simulink model "ICAES_R2025aa_real_a"  (R2025a)
settings: Solver=FixedStepAuto  StartTime=0.0  StopTime=stopt  FixedStep=deltat  MaxStep=0.05  RelTol=1e-3
InitFcn:
  | clear all;
  | close all;
  | clc;
  | 
  | % add the data and script directories
  | addpath('data','scripts');
  | 
  | % load the constants (units)
  | constants;
  | 
  | % load the simulation parameters
  | preprocessing;
StopFcn:
  | postprocessing;
values from neighbouring files (symbols this model uses):
  c_p = 1005    [icaes_parameter_sweep.m]    (also in preprocessing.m = 1005 * unit("J") / (unit("kg") * unit("K")))
  c_tes = 4184    [icaes_parameter_sweep.m]    (also in preprocessing.m = 4184 * unit("J") / (unit("kg") * unit("K")))
  eta_comp = 0.833    [icaes_parameter_sweep.m]    (also in preprocessing.m)
  eta_exp = 0.85    [icaes_parameter_sweep.m]    (also in preprocessing.m)
  m_tes = m_tes_range(im)    [icaes_parameter_sweep.m]    (also in preprocessing.m = 5000000 * unit("kg"))
  n_poly = 1.1    [icaes_parameter_sweep.m]    (also in preprocessing.m)
  p_amb = 101325    [icaes_parameter_sweep.m]    (also in preprocessing.m = 101325 * unit("Pa"))
  P_limit = 300e6    (= 300000000)    [icaes_parameter_sweep.m]    (also in preprocessing.m = 300 * unit("MW"))
  p_store_max = 100e5    (= 10000000)    [icaes_parameter_sweep.m]    (also in preprocessing.m = 80 * unit("bar"))
  R_air = 287.05    [icaes_parameter_sweep.m]    (also in preprocessing.m = 287.05 * unit("J") / (unit("kg") * unit("K")))
  T_amb = 300    [icaes_parameter_sweep.m]    (also in preprocessing.m = 300 * unit("K"))
  T_tes_initial = T_amb    [preprocessing.m]
  V_cavern = V_cav_range(iv)    [icaes_parameter_sweep.m]    (also in preprocessing.m = 310000 * unit("m^3"))
undefined symbols (not defined in the file or in its folder): Cablelength, Cablevoltage, m_air_initial, m_air_max, mdot_max, Rprime, T_expand, T_tes_max
settings Model: Creator=joche  LastModifiedBy=ASUS
settings DataIOCC: SaveFormat=Array  SaveOutput=off  ReturnWorkspaceOutputs=off
settings OptimizationCC: ReuseModelBlockBuffer=off
settings ModelReferenceCC: EnableRefExpFcnMdlSchedulingChecks=on
settings RTWCC: GPUComputeCapability=3.5

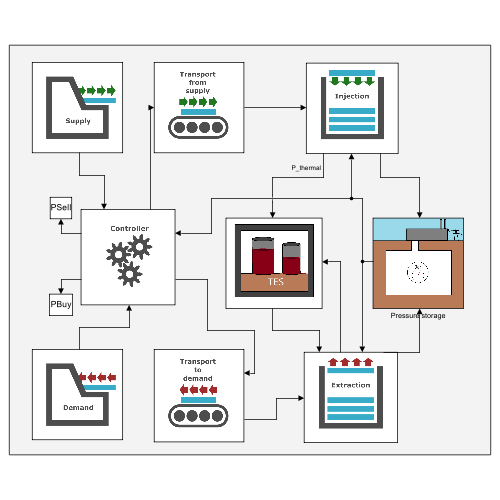
[thumbnail: Simulink's stored preview of the top-level diagram]
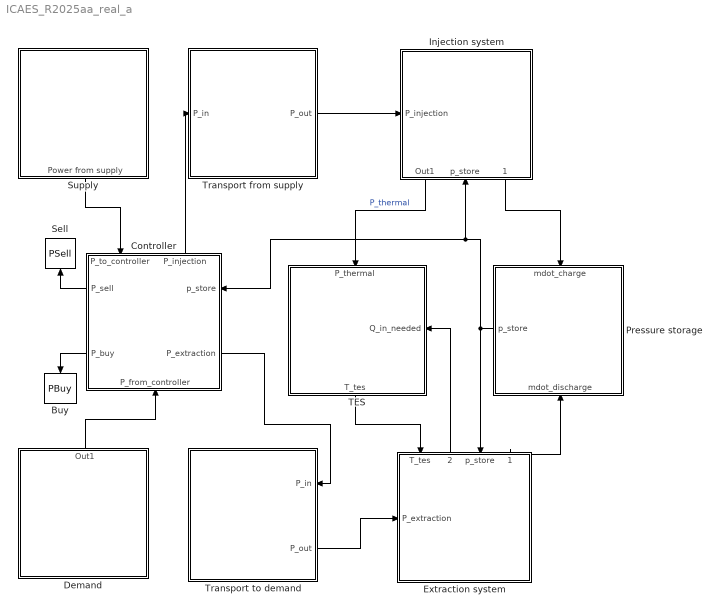
== system ICAES_R2025aa_real_a ==
  Buy : ToWorkspace  VariableName=PBuy  SampleTime=-1
  Controller : Subsystem
      settings: PortSchema="{\"entries\":[{\"content\":{\"sides\":[{\"content\":{\"connectorIds\":[\"Out3\",\"Out4\"]},\"type\":\"ConnectorPlacement.EquallySpacedRectSide\",\"uuid\":\"4daf33ce-c96a-4783-b5c4-228eed953e01\"},{\"content\":{\"connectorIds\":[\"In3\",\"Out1\"],\"side\":\"RIGHT\"},\"type\":\"ConnectorPlacement.EquallySpacedRectSide\",\"uuid\":\"e9942e50-8467-4af8-b79b-80636cbc76e5\"},{\"content\":{\"connectorIds\":[\"In1\",\"Out2\"],\"side\":\"TOP\"},\"type\":\"ConnectorPlacement.EquallySpacedRectSide\",\"uuid\":\"f315e931-d69b-4751-b712-f89c6c81baeb\"},{\"content\":{\"connectorIds\":[\"In2\"],\"side\":\"BOTTOM\"},\"type\":\"ConnectorPlacement.EquallySpacedRectSide\",\"uuid\":\"44715ee6-5cd5-4669-bcb9-5ed7c869bdb3\"}]},\"type\":\"ConnectorPlacement.EquallySpacedConnector\",\"uuid\":\"fff48899-944b-4064-b7d7-ecc12144fb48\"}],\"packageUris\":[\"http://schema.mathworks.com/mf0/Connector/R2020b\"],\"version\":\"1.0\"}"
      mask Display: image('$imagefile'); % Use "Edit Image" on toolstrip to change.
  Demand : Subsystem
      settings: PortSchema="{\"entries\":[{\"content\":{\"sides\":[{\"content\":{},\"type\":\"ConnectorPlacement.EquallySpacedRectSide\",\"uuid\":\"f27962e9-c4d7-4452-9990-e0f79d5e43d2\"},{\"content\":{\"side\":\"RIGHT\"},\"type\":\"ConnectorPlacement.EquallySpacedRectSide\",\"uuid\":\"2b278ec5-7432-4b51-af5a-f36413392bbe\"},{\"content\":{\"connectorIds\":[\"Out1\"],\"side\":\"TOP\"},\"type\":\"ConnectorPlacement.EquallySpacedRectSide\",\"uuid\":\"4ad1aacd-5412-446e-ba31-db0d1d02529a\"}]},\"type\":\"ConnectorPlacement.EquallySpacedConnector\",\"uuid\":\"5190d484-8789-4ab4-af36-e8ecab949163\"}],\"packageUris\":[\"http://schema.mathworks.com/mf0/Connector/R2020b\"],\"version\":\"1.0\"}"
      mask Display: image('$imagefile'); % Use "Edit Image" on toolstrip to change.
  Extraction system : Subsystem
      settings: PortSchema="{\"entries\":[{\"content\":{\"sides\":[{\"content\":{},\"type\":\"ConnectorPlacement.EquallySpacedRectSide\",\"uuid\":\"05c5933d-55fc-4e06-853f-fc26d42905f9\"},{\"content\":{\"connectorIds\":[\"In3\"],\"side\":\"RIGHT\"},\"type\":\"ConnectorPlacement.EquallySpacedRectSide\",\"uuid\":\"327426c5-31d5-498b-a2bd-83e49353408c\"},{\"content\":{\"side\":\"TOP\"},\"type\":\"ConnectorPlacement.EquallySpacedRectSide\",\"uuid\":\"55306cf3-a3de-4385-a5ae-b8600ecdd5a2\"},{\"content\":{\"connectorIds\":[\"Out1\",\"In1\",\"Out2\",\"In2\"],\"side\":\"BOTTOM\"},\"type\":\"ConnectorPlacement.EquallySpacedRectSide\",\"uuid\":\"08fcc9c3-40d3-4ac6-b914-dfeef6039ffb\"}]},\"type\":\"ConnectorPlacement.EquallySpacedConnector\",\"uuid\":\"cb35d5ba-e8c6-462c-b7b2-fe8356d4b0a1\"}],\"packageUris\":[\"http://schema.mathworks.com/mf0/Connector/R2020b\"],\"version\":\"1.0\"}"
      mask Display: image('$imagefile'); % Use "Edit Image" on toolstrip to change.
  Injection system : Subsystem
      settings: PortSchema="{\"entries\":[{\"content\":{\"sides\":[{\"content\":{},\"type\":\"ConnectorPlacement.EquallySpacedRectSide\",\"uuid\":\"05c5933d-55fc-4e06-853f-fc26d42905f9\"},{\"content\":{\"connectorIds\":[\"In2\"],\"side\":\"RIGHT\"},\"type\":\"ConnectorPlacement.EquallySpacedRectSide\",\"uuid\":\"327426c5-31d5-498b-a2bd-83e49353408c\"},{\"content\":{\"connectorIds\":[\"Out1\",\"In1\",\"Out2\"],\"side\":\"TOP\"},\"type\":\"ConnectorPlacement.EquallySpacedRectSide\",\"uuid\":\"55306cf3-a3de-4385-a5ae-b8600ecdd5a2\"},{\"content\":{\"side\":\"BOTTOM\"},\"type\":\"ConnectorPlacement.EquallySpacedRectSide\",\"uuid\":\"08fcc9c3-40d3-4ac6-b914-dfeef6039ffb\"}]},\"type\":\"ConnectorPlacement.EquallySpacedConnector\",\"uuid\":\"cb35d5ba-e8c6-462c-b7b2-fe8356d4b0a1\"}],\"packageUris\":[\"http://schema.mathworks.com/mf0/Connector/R2020b\"],\"version\":\"1.0\"}"
      mask Display: image('$imagefile'); % Use "Edit Image" on toolstrip to change.
  Pressure storage : Subsystem
      settings: PortSchema="{\"entries\":[{\"content\":{\"sides\":[{\"content\":{\"connectorIds\":[\"Out1\"]},\"type\":\"ConnectorPlacement.EquallySpacedRectSide\",\"uuid\":\"d889665d-bfbe-4c74-9411-d83433156a63\"},{\"content\":{\"side\":\"RIGHT\"},\"type\":\"ConnectorPlacement.EquallySpacedRectSide\",\"uuid\":\"048dbb4a-051e-49bc-807c-40b31b00f8e2\"},{\"content\":{\"connectorIds\":[\"In1\"],\"side\":\"TOP\"},\"type\":\"ConnectorPlacement.EquallySpacedRectSide\",\"uuid\":\"a4af44e9-b107-4f3e-88f5-e97fca389ca7\"},{\"content\":{\"connectorIds\":[\"In2\"],\"side\":\"BOTTOM\"},\"type\":\"ConnectorPlacement.EquallySpacedRectSide\",\"uuid\":\"8e783e88-b9a1-4588-afaa-b223ffbcf4c7\"}]},\"type\":\"ConnectorPlacement.EquallySpacedConnector\",\"uuid\":\"03b1cead-97d2-49f0-bef1-8cdb04da0e6d\"}],\"packageUris\":[\"http://schema.mathworks.com/mf0/Connector/R2020b\"],\"version\":\"1.0\"}"
      mask Display: image('pressure storage.png');
  Sell : ToWorkspace  VariableName=PSell  SampleTime=-1
  Supply : Subsystem
      settings: PortSchema="{\"entries\":[{\"content\":{\"sides\":[{\"content\":{},\"type\":\"ConnectorPlacement.EquallySpacedRectSide\",\"uuid\":\"f27962e9-c4d7-4452-9990-e0f79d5e43d2\"},{\"content\":{\"side\":\"RIGHT\"},\"type\":\"ConnectorPlacement.EquallySpacedRectSide\",\"uuid\":\"2b278ec5-7432-4b51-af5a-f36413392bbe\"},{\"content\":{\"side\":\"TOP\"},\"type\":\"ConnectorPlacement.EquallySpacedRectSide\",\"uuid\":\"4ad1aacd-5412-446e-ba31-db0d1d02529a\"},{\"content\":{\"connectorIds\":[\"Out1\"],\"side\":\"BOTTOM\"},\"type\":\"ConnectorPlacement.EquallySpacedRectSide\",\"uuid\":\"c559864b-71ed-434e-b1c1-5c3f122c4164\"}]},\"type\":\"ConnectorPlacement.EquallySpacedConnector\",\"uuid\":\"5190d484-8789-4ab4-af36-e8ecab949163\"}],\"packageUris\":[\"http://schema.mathworks.com/mf0/Connector/R2020b\"],\"version\":\"1.0\"}"
      mask Display: image('$imagefile'); % Use "Edit Image" on toolstrip to change.
  TES : Subsystem
      settings: PortSchema="{\"entries\":[{\"content\":{\"sides\":[{\"content\":{},\"type\":\"ConnectorPlacement.EquallySpacedRectSide\",\"uuid\":\"d889665d-bfbe-4c74-9411-d83433156a63\"},{\"content\":{\"connectorIds\":[\"In2\"],\"side\":\"RIGHT\"},\"type\":\"ConnectorPlacement.EquallySpacedRectSide\",\"uuid\":\"048dbb4a-051e-49bc-807c-40b31b00f8e2\"},{\"content\":{\"connectorIds\":[\"In1\"],\"side\":\"TOP\"},\"type\":\"ConnectorPlacement.EquallySpacedRectSide\",\"uuid\":\"a4af44e9-b107-4f3e-88f5-e97fca389ca7\"},{\"content\":{\"connectorIds\":[\"Out1\"],\"side\":\"BOTTOM\"},\"type\":\"ConnectorPlacement.EquallySpacedRectSide\",\"uuid\":\"12f882ff-043d-4bf9-a0d2-8249dbdd2f93\"}]},\"type\":\"ConnectorPlacement.EquallySpacedConnector\",\"uuid\":\"03b1cead-97d2-49f0-bef1-8cdb04da0e6d\"}],\"packageUris\":[\"http://schema.mathworks.com/mf0/Connector/R2020b\"],\"version\":\"1.0\"}"
      mask Display: image('TES_image.png');
  Transport from supply : Subsystem
      mask Display: image('$imagefile'); % Use "Edit Image" on toolstrip to change.
  Transport to demand : Subsystem
      settings: PortSchema="{\"entries\":[{\"content\":{\"sides\":[{\"content\":{},\"type\":\"ConnectorPlacement.EquallySpacedRectSide\",\"uuid\":\"5f97e25a-2218-4bfd-a92e-89da500073ba\"},{\"content\":{\"connectorIds\":[\"In1\",\"Out1\"],\"side\":\"RIGHT\"},\"type\":\"ConnectorPlacement.EquallySpacedRectSide\",\"uuid\":\"57326547-f9ab-4d29-843f-dcc54e723c8b\"},{\"content\":{\"side\":\"TOP\"},\"type\":\"ConnectorPlacement.EquallySpacedRectSide\",\"uuid\":\"3bb3598b-01a5-470c-8e1a-4dd11c24bba5\"}]},\"type\":\"ConnectorPlacement.EquallySpacedConnector\",\"uuid\":\"eb6225b8-aa64-4044-a8a8-f6e209634de3\"}],\"packageUris\":[\"http://schema.mathworks.com/mf0/Connector/R2020b\"],\"version\":\"1.0\"}"
      mask Display: image('$imagefile'); % Use "Edit Image" on toolstrip to change.
  wires:
  Controller/3(P_sell) -> Sell/1
  Controller/1(P_extraction) -> Transport to demand/1(P_in)
  Controller/4(P_buy) -> Buy/1
  Pressure storage/1(p_store) -> Controller/3(p_store), Injection system/1(p_store), Extraction system/1(p_store)
  Injection system/2(Out1) -> TES/1(P_thermal)  "P_thermal"
  Extraction system/2(Q_in_needed) -> TES/2(Q_in_needed)
  TES/1(T_tes) -> Extraction system/2(T_tes)
  Supply/1(Power from supply) -> Controller/1(P_to_controller)
  Demand/1(Out1) -> Controller/2(P_from_controller)
  Extraction system/1(mdot_discharge) -> Pressure storage/2(mdot_discharge)
  Injection system/1(mdot_charge) -> Pressure storage/1(mdot_charge)
  Controller/2(P_injection) -> Transport from supply/1(P_in)
  Transport from supply/1(P_out) -> Injection system/2(P_injection)
  Transport to demand/1(P_out) -> Extraction system/3(P_extraction)

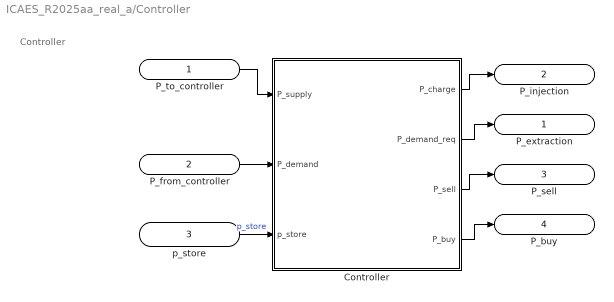
== system ICAES_R2025aa_real_a/Controller ==
  note: Controller
  P_to_controller : Inport
  P_from_controller : Inport  Port=2
  p_store : Inport  Port=3
  Controller : MATLAB Function  TreatAsAtomicUnit=on
  P_extraction : Outport
  P_injection : Outport  Port=2
  P_sell : Outport  Port=3
  P_buy : Outport  Port=4
  wires:
  P_from_controller/1 -> Controller/2(P_demand)
  Controller/2(P_demand_req) -> P_extraction/1
  Controller/3(P_sell) -> P_sell/1
  Controller/4(P_buy) -> P_buy/1
  P_to_controller/1 -> Controller/1(P_supply)
  Controller/1(P_charge) -> P_injection/1
  p_store/1 -> Controller/3(p_store)  "p_store"

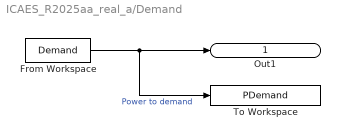
== system ICAES_R2025aa_real_a/Demand ==
  From Workspace : FromWorkspace  VariableName=Demand  OutputAfterFinalValue=Setting to zero
  To Workspace : ToWorkspace  VariableName=PDemand  SampleTime=-1
  Out1 : Outport
  wires:
  From Workspace/1 -> To Workspace/1, Out1/1  "Power to demand"

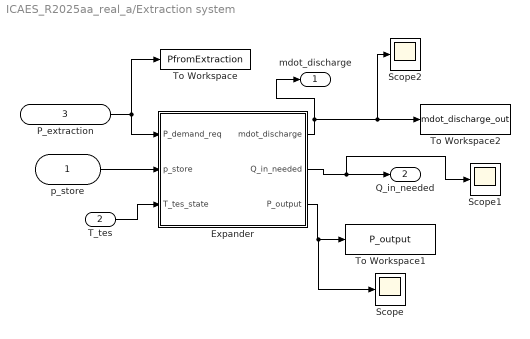
== system ICAES_R2025aa_real_a/Extraction system ==
  p_store : Inport
  T_tes : Inport  Port=2
  P_extraction : Inport  Port=3
  Expander : MATLAB Function  TreatAsAtomicUnit=on
  Scope : Scope
      settings: ActiveDisplayYMinimum=-1  ActiveDisplayYMaximum=1  DataLoggingVariableName=ScopeData2
  Scope1 : Scope
      settings: ActiveDisplayYMinimum=-1  ActiveDisplayYMaximum=1  DataLoggingVariableName=ScopeData3
  Scope2 : Scope
      settings: ActiveDisplayYMinimum=-1143.2890833418655  ActiveDisplayYMaximum=10289.601750076792  DataLoggingVariableName=ScopeData5
  To Workspace : ToWorkspace  VariableName=PfromExtraction  SampleTime=-1
  To Workspace1 : ToWorkspace  VariableName=P_output  SampleTime=-1
  To Workspace2 : ToWorkspace  VariableName=mdot_discharge_out  SampleTime=-1
  mdot_discharge : Outport
  Q_in_needed : Outport  Port=2
  wires:
  P_extraction/1 -> To Workspace/1, Expander/1(P_demand_req)
  p_store/1 -> Expander/2(p_store)
  Expander/3(P_output) -> Scope/1, To Workspace1/1
  Expander/2(Q_in_needed) -> Scope1/1, Q_in_needed/1
  T_tes/1 -> Expander/3(T_tes_state)
  Expander/1(mdot_discharge) -> mdot_discharge/1, Scope2/1, To Workspace2/1

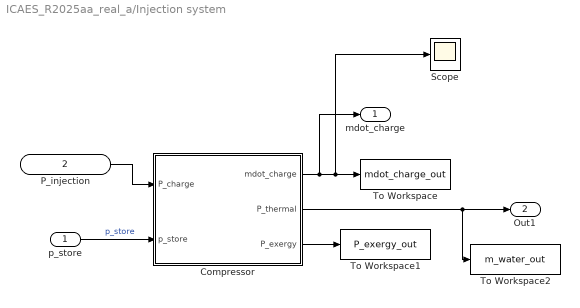
== system ICAES_R2025aa_real_a/Injection system ==
  p_store : Inport
  P_injection : Inport  Port=2
  Compressor : MATLAB Function  TreatAsAtomicUnit=on
  Scope : Scope
      settings: ActiveDisplayYMinimum=-3019.24635169851  ActiveDisplayYMaximum=27173.217165286616  DataLoggingVariableName=ScopeData4
  To Workspace : ToWorkspace  VariableName=mdot_charge_out  SampleTime=-1
  To Workspace1 : ToWorkspace  VariableName=P_exergy_out  SampleTime=-1
  To Workspace2 : ToWorkspace  VariableName=m_water_out  SampleTime=-1
  mdot_charge : Outport
  Out1 : Outport  Port=2
  wires:
  P_injection/1 -> Compressor/1(P_charge)
  p_store/1 -> Compressor/2(p_store)  "p_store"
  Compressor/2(P_thermal) -> To Workspace2/1, Out1/1
  Compressor/3(P_exergy) -> To Workspace1/1
  Compressor/1(mdot_charge) -> mdot_charge/1, Scope/1, To Workspace/1

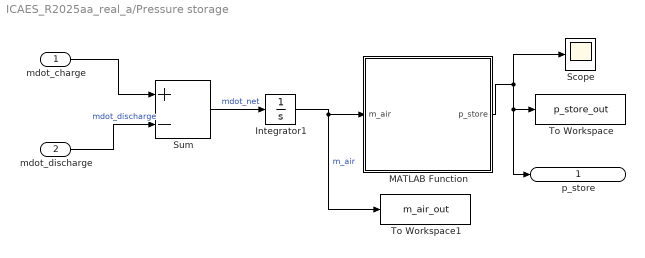
== system ICAES_R2025aa_real_a/Pressure storage ==
  mdot_charge : Inport
  mdot_discharge : Inport  Port=2
  Integrator1 : Integrator  InitialCondition=m_air_initial  LimitOutput=on  UpperSaturationLimit=m_air_max  LowerSaturationLimit=0
  MATLAB Function : MATLAB Function  TreatAsAtomicUnit=on
  Scope : Scope
      settings: ActiveDisplayYMinimum=-2.2901277573217703E+6  ActiveDisplayYMaximum=1.1403864273455586E+7
  Sum : Sum  Inputs=+-
  To Workspace : ToWorkspace  VariableName=p_store_out  SampleTime=-1
  To Workspace1 : ToWorkspace  VariableName=m_air_out  SaveFormat=Timeseries  SampleTime=-1
  p_store : Outport
  wires:
  mdot_discharge/1 -> Sum/2  "mdot_discharge"
  mdot_charge/1 -> Sum/1
  Sum/1 -> Integrator1/1  "mdot_net"
  Integrator1/1 -> To Workspace1/1, MATLAB Function/1(m_air)  "m_air"
  MATLAB Function/1(p_store) -> Scope/1, p_store/1, To Workspace/1

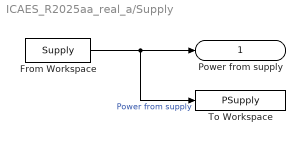
== system ICAES_R2025aa_real_a/Supply ==
  From Workspace : FromWorkspace  VariableName=Supply  OutputAfterFinalValue=Setting to zero
  To Workspace : ToWorkspace  VariableName=PSupply  SampleTime=-1
  Power from supply : Outport
  wires:
  From Workspace/1 -> To Workspace/1, Power from supply/1  "Power from supply"

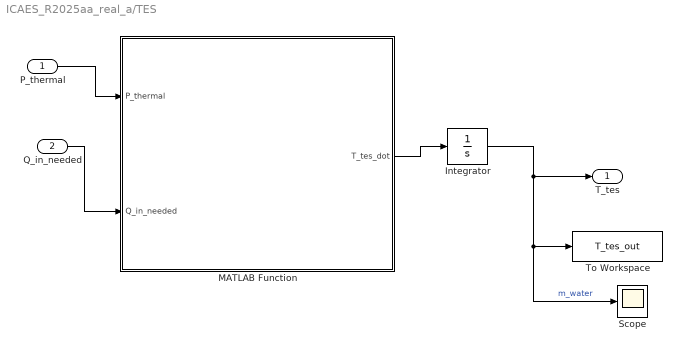
== system ICAES_R2025aa_real_a/TES ==
  P_thermal : Inport
  Q_in_needed : Inport  Port=2
  Integrator : Integrator  InitialCondition=T_tes_initial  LimitOutput=on  UpperSaturationLimit=T_tes_max  LowerSaturationLimit=T_amb
  MATLAB Function : MATLAB Function  TreatAsAtomicUnit=on
  Scope : Scope
      settings: ActiveDisplayYMinimum=-1  ActiveDisplayYMaximum=1
  To Workspace : ToWorkspace  VariableName=T_tes_out  SampleTime=-1
  T_tes : Outport
  wires:
  P_thermal/1 -> MATLAB Function/1(P_thermal)
  Q_in_needed/1 -> MATLAB Function/2(Q_in_needed)
  MATLAB Function/1(T_tes_dot) -> Integrator/1
  Integrator/1 -> T_tes/1, Scope/1, To Workspace/1  "m_water"

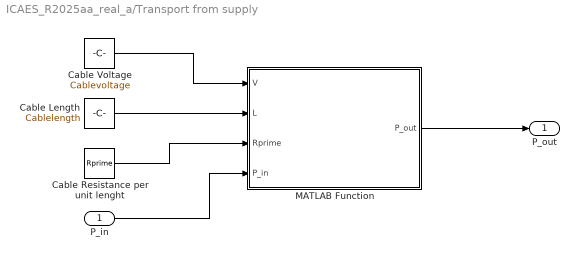
== system ICAES_R2025aa_real_a/Transport from supply ==
  P_in : Inport
  Cable Length : Constant  Value=Cablelength
  Cable Resistance per unit lenght : Constant  Value=Rprime
  Cable Voltage : Constant  Value=Cablevoltage
  MATLAB Function : MATLAB Function  TreatAsAtomicUnit=on
  P_out : Outport
  wires:
  P_in/1 -> MATLAB Function/4(P_in)
  MATLAB Function/1(P_out) -> P_out/1
  Cable Resistance per unit lenght/1 -> MATLAB Function/3(Rprime)
  Cable Length/1 -> MATLAB Function/2(L)
  Cable Voltage/1 -> MATLAB Function/1(V)

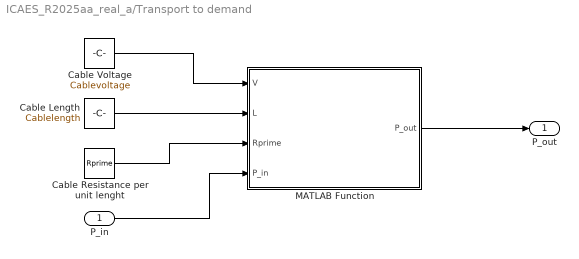
== system ICAES_R2025aa_real_a/Transport to demand ==
  P_in : Inport
  Cable Length : Constant  Value=Cablelength
  Cable Resistance per unit lenght : Constant  Value=Rprime
  Cable Voltage : Constant  Value=Cablevoltage
  MATLAB Function : MATLAB Function  TreatAsAtomicUnit=on
  P_out : Outport
  wires:
  Cable Voltage/1 -> MATLAB Function/1(V)
  Cable Length/1 -> MATLAB Function/2(L)
  MATLAB Function/1(P_out) -> P_out/1
  P_in/1 -> MATLAB Function/4(P_in)
  Cable Resistance per unit lenght/1 -> MATLAB Function/3(Rprime)

== matlab function ICAES_R2025aa_real_a/Transport from supply/MATLAB Function ==
  data: P_out output; V input; L input; Rprime input; P_in input
function P_out = Transport_from_supply(V,L,Rprime, P_in)

P_out = (1-L*Rprime*P_in/V^2)*P_in;

== matlab function ICAES_R2025aa_real_a/Transport to demand/MATLAB Function ==
  data: P_out output; V input; L input; Rprime input; P_in input
function P_out = Transport_to_demand(V,L,Rprime, P_in)

P_out = (1-L*Rprime*P_in/V^2)*P_in;

== matlab function ICAES_R2025aa_real_a/Injection system/Compressor ==
  data: P_charge input; mdot_charge output; p_store input; P_thermal output; P_exergy output; eta_comp parameter; n_poly parameter; R_air parameter; c_p parameter; T_amb parameter; p_amb parameter; mdot_max parameter
function [mdot_charge, P_thermal, P_exergy] = compressor( ...
    P_charge, p_store, ...
    eta_comp, n_poly, R_air, c_p, T_amb, p_amb, mdot_max)
%COMPRESSOR  Polytropic compression with pipe flow limit.
%   Converts electrical power into thermal energy (→TES) and
%   pressure exergy (→Cavern) via mass flow of compressed air.
%   mdot_charge is capped at mdot_max (physical pipe capacity ρ·A·v_max).
%
%   Equations from model: (2.8), (2.9), (2.10), (2.11)

    mdot_charge = 0;
    P_thermal   = 0;
    P_exergy    = 0;

    if P_charge <= 0
        return;
    end

    % Pressure ratio
    ratio = p_store / p_amb;
    if ratio <= 1
        ratio = 1.001;  % Guard: cavern at ambient
    end

    % Polytropic specific work [J/kg]  — Eq. 2.8
    poly_factor = (n_poly/(n_poly-1)) * R_air * T_amb * (ratio^((n_poly-1)/n_poly) - 1);

    % Thermodynamic mass flow rate [kg/s]  — Eq. 2.9
    mdot_charge = P_charge / (eta_comp * poly_factor);

    % Apply physical pipe flow limit [kg/s]
    mdot_charge = min(mdot_charge, mdot_max);

    % Actual electrical power consumed after flow cap [W]
    % (may be < P_charge when pipe is the bottleneck)
    P_used = mdot_charge * eta_comp * poly_factor;

    % Compressor outlet temperature [K]
    T_out = T_amb * ratio^((n_poly-1)/n_poly);

    % Thermal power delivered to TES [W]  — Eq. 2.10
    P_thermal = P_used - mdot_charge * c_p * (T_out - T_amb);
    if P_thermal < 0
        P_thermal = 0;  % Guard
    end

    % Pressure exergy rate stored in cavern [W]  — Eq. 2.11
    P_exergy = mdot_charge * R_air * T_amb * log(ratio);
end

== matlab function ICAES_R2025aa_real_a/Pressure storage/MATLAB Function ==
  data: m_air input; p_store output; R_air parameter; T_amb parameter; V_cavern parameter
function p_store = equation_of_state(m_air, R_air, T_amb, V_cavern)
%EQUATION_OF_STATE  Ideal gas law: compute pressure from mass.
%   p = m * R * T / V

    p_store = m_air * R_air * T_amb / V_cavern;
end

== matlab function ICAES_R2025aa_real_a/Controller/Controller ==
  data: P_charge output; P_demand_req output; P_sell output; P_buy output; P_supply input; P_demand input; p_store input; P_limit parameter; p_store_max parameter; p_amb parameter
function [P_charge, P_demand_req, P_sell, P_buy] = controller( ...
    P_supply, P_demand, p_store, ...
    P_limit, p_store_max, p_amb)
%CONTROLLER  Determines charging/discharging mode based on P_net.
%   P_net >= 0  →  charge (compress air)
%   P_net <  0  →  discharge (expand air)
%
%   NOTE: eta_tran is now handled by the Transport blocks, not here.

    P_net = P_supply - P_demand;

    % Default outputs
    P_charge = 0;
    P_demand_req = 0;
    P_sell = 0;
    P_buy = 0;

    if P_net >= 0
        % === CHARGING MODE ===
        P_available = min(P_net, P_limit);
        P_charge = P_available;               % NO eta_tran here anymore
        P_sell = (P_net - P_available);       % Excess beyond P_limit

        % Stop charging if cavern full
        if p_store >= p_store_max
            P_sell = P_sell + P_charge;
            P_charge = 0;
        end
    else
        % === DISCHARGING MODE ===
        P_demand_req = -P_net;                % Positive value

        % Stop discharging if cavern nearly empty
        if p_store <= p_amb * 1.05
            P_buy = P_demand_req;
            P_demand_req = 0;
        end
    end
end

== matlab function ICAES_R2025aa_real_a/Extraction system/Expander ==
  data: P_demand_req input; mdot_discharge output; p_store input; T_tes_state input; eta_exp parameter; n_poly parameter; R_air parameter; c_p parameter; p_amb parameter; Q_in_needed output; P_output output; T_amb parameter; T_expand parameter; mdot_max parameter
function [mdot_discharge, Q_in_needed, P_output] = expander( ...
    P_demand_req, p_store, T_tes_state, ...
    eta_exp, n_poly, R_air, c_p, p_amb, T_amb, T_expand, mdot_max)
%EXPANDER  Polytropic expansion with dynamic mode selection and pipe flow limit.
%   When TES is hot enough (T_tes_state >= T_expand): near-isothermal (n = n_poly)
%   When TES is cold: adiabatic (n = gamma)
%   mdot_discharge is capped at mdot_max (physical pipe capacity ρ·A·v_max).
%   If flow-limited, P_output < P_demand_req (demand is partially unmet).
%
%   NOTE: eta_tran is handled by the Transport blocks, not here.

    mdot_discharge = 0;
    Q_in_needed    = 0;
    P_output       = 0;

    if P_demand_req <= 0
        return;
    end

    % Pressure ratio (expansion direction: p_amb/p_store < 1)
    ratio = p_amb / p_store;
    if ratio >= 1
        return;
    end

    gamma = c_p / (c_p - R_air);

    if T_tes_state >= T_expand
        n    = n_poly;
        T_in = T_expand;
    else
        n    = gamma;
        T_in = T_amb;
    end

    % Polytropic expansion specific work [J/kg]
    poly_factor = (n/(n-1)) * R_air * T_in * (1 - ratio^((n-1)/n));

    if poly_factor <= 0
        return;
    end

    % Thermodynamic mass flow rate [kg/s]
    mdot_discharge = P_demand_req / (eta_exp * poly_factor);

    % Apply physical pipe flow limit [kg/s]
    mdot_discharge = min(mdot_discharge, mdot_max);

    % Expander outlet temperature [K]
    T_out = T_in * ratio^((n-1)/n);

    % Actual mechanical power output after flow cap [W]
    % (may be < P_demand_req when pipe is the bottleneck)
    P_output = mdot_discharge * eta_exp * poly_factor;

    % Thermal power drawn from TES [W]
    if T_tes_state >= T_expand
        Q_in_needed = P_output / eta_exp - mdot_discharge * c_p * (T_in - T_out);
        if Q_in_needed < 0
            Q_in_needed = 0;
        end
    else
        Q_in_needed = 0;
    end
end

== matlab function ICAES_R2025aa_real_a/TES/MATLAB Function ==
  data: P_thermal input; T_tes_dot output; Q_in_needed input; m_tes parameter; c_tes parameter
function T_tes_dot = tes_dynamics(P_thermal, Q_in_needed, m_tes, c_tes)
%TES_DYNAMICS  Fixed-mass, variable-temperature salt bed TES.
%   Salt bed mass is constant. Temperature rises when charging,
%   falls when discharging.
%
%   dT/dt = (Q_in - Q_out) / (m_tes * c_tes)

    % Thermal capacitance of the salt bed [J/K]
    C_tes = m_tes * c_tes;

    % Rate of temperature change [K/s]
    T_tes_dot = (P_thermal - Q_in_needed) / C_tes;
end
